simulink library "CAN_out_lib"  (R2016b)
settings: Solver=VariableStepAuto  StartTime=0.0  StopTime=10.0  RelTol=1e-3
undefined symbols (not defined in the file): body_rates, fsw_params, point_true, sc_above_gs, sc_mode, sc_quat
libraries: bus_stubs_fsw x1, quat_degerr_check x1
settings Model: Creator=taylorreynolds  LastModifiedBy=Taylor

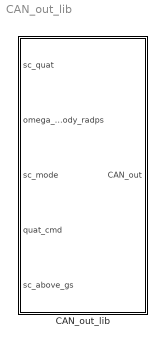
== system CAN_out_lib ==
  CAN_out_lib : Subsystem

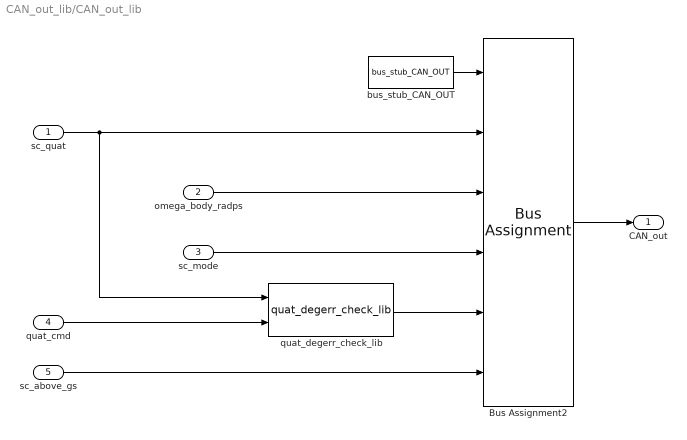
== system CAN_out_lib/CAN_out_lib ==
  sc_quat : Inport
  omega_body_radps : Inport  Port=2
  sc_mode : Inport  Port=3
  quat_cmd : Inport  Port=4
  sc_above_gs : Inport  Port=5
  Bus Assignment2 : BusAssignment  AssignedSignals=sc_quat,body_rates,sc_mode,point_true,sc_above_gs
  bus_stub_CAN_OUT : bus_stubs_fsw/bus_stub_CAN_OUT
  quat_degerr_check_lib : quat_degerr_check/quat_degerr_check_lib  const=fsw_params.bus.point_tol
  CAN_out : Outport
  wires:
  bus_stub_CAN_OUT/1 -> Bus Assignment2/1
  Bus Assignment2/1 -> CAN_out/1
  sc_quat/1 -> Bus Assignment2/2, quat_degerr_check_lib/1
  omega_body_radps/1 -> Bus Assignment2/3
  sc_mode/1 -> Bus Assignment2/4
  quat_cmd/1 -> quat_degerr_check_lib/2
  quat_degerr_check_lib/1 -> Bus Assignment2/5
  sc_above_gs/1 -> Bus Assignment2/6
